simulink model "example_sdofplant"  (R2022b)
settings: Solver=VariableStepAuto  StartTime=0.0  StopTime=10.0  RelTol=1e-3
model workspace: external: MATLAB File exmaple_initdata.m (data not in the file)
undefined symbols (not defined in the file or in its folder): convertTo, datetime, Earth, F, Light, MIL, WGS84, WMM2020
libraries: aerolibconvert2 x5, aerolibasang x5, aerolibactuator x3, aerolibwind2 x3, aerolib6dof2 x1, aerolibatmos2 x1, aerolibgravity2 x1
settings Model: DataDictionary=example.sldd  Creator=zhanfuyu  LastModifiedBy=CETCA

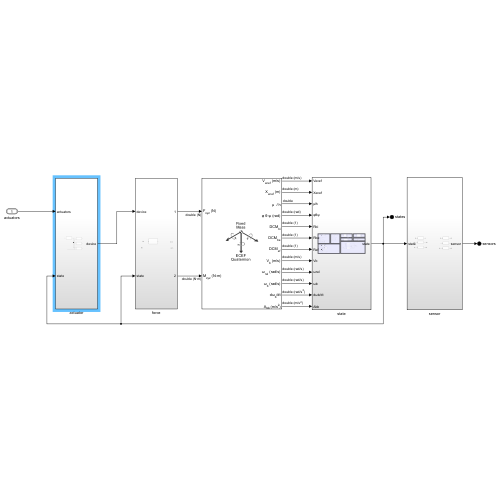
[thumbnail: Simulink's stored preview of the top-level diagram]
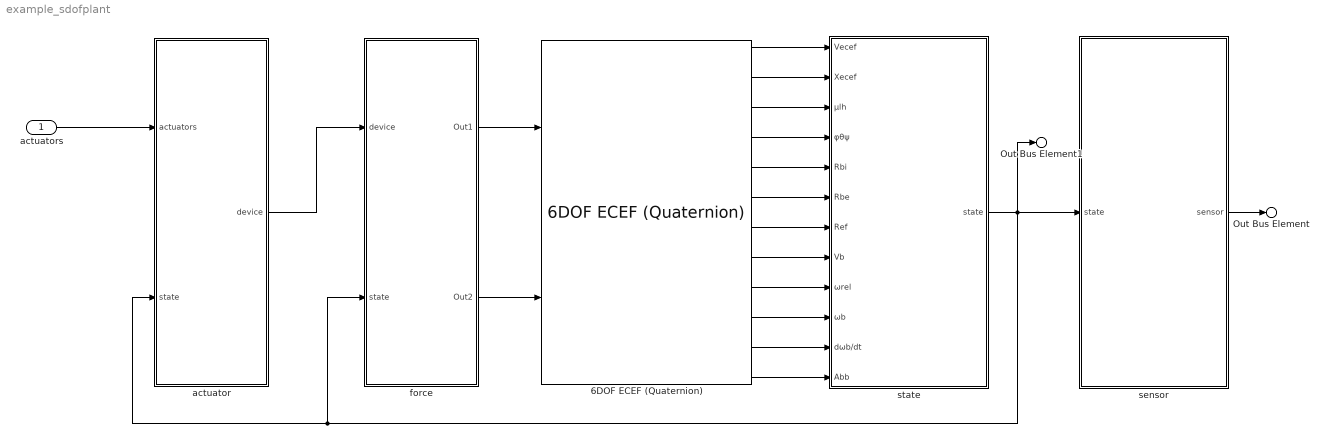
== system example_sdofplant ==
  actuators : Inport  OutDataTypeStr=Bus: actuator_outputs_s
  6DOF ECEF (Quaternion) : aerolib6dof2/6DOF ECEF (Quaternion)  units=Metric (MKS)  mtype=Fixed  xg_0=[0 0 0]  Vm_0=[0 0 0]  eul_0=[0 0 0]  pm_0=[0 0 0]  mass_0=1.0  mass_e=0.5  mass_f=2.0  inertia=eye(3)  inertia_e=eye(3)  inertia_f=2*eye(3)  vre_flag=on  abi_flag=off  ptype=Earth (WGS84)  R=6378137  F=1/298.257223563  w_E=7292115e-11  angle_in=Internal  LG0=0  quat_statename=''  pm_statename=''  Vm_statename=''  posECEF_statename=''  posECI_statename=''  LG_statename=''  mass_statename=''
  actuator : Subsystem
  force : Subsystem
  sensor : Subsystem
  state : Subsystem
  Out Bus Element : Outport  PortName=sensors
  Out Bus Element1 : Outport  Port=2  PortName=states
  wires:
  6DOF ECEF (Quaternion)/1 -> state/1(Vecef)
  6DOF ECEF (Quaternion)/2 -> state/2(Xecef)
  6DOF ECEF (Quaternion)/3 -> state/3(μlh)
  6DOF ECEF (Quaternion)/4 -> state/4(φθψ)
  6DOF ECEF (Quaternion)/5 -> state/5(Rbi)
  6DOF ECEF (Quaternion)/6 -> state/6(Rbe)
  6DOF ECEF (Quaternion)/7 -> state/7(Ref)
  6DOF ECEF (Quaternion)/8 -> state/8(Vb)
  6DOF ECEF (Quaternion)/9 -> state/9(ωrel)
  6DOF ECEF (Quaternion)/10 -> state/10(ωb)
  6DOF ECEF (Quaternion)/11 -> state/11(dωb/dt)
  6DOF ECEF (Quaternion)/12 -> state/12(Abb)
  state/1(state) -> Out Bus Element1/1, force/2(state), actuator/2(state), sensor/1(state)
  sensor/1(sensor) -> Out Bus Element/1
  force/1(Out1) -> 6DOF ECEF (Quaternion)/1
  force/2(Out2) -> 6DOF ECEF (Quaternion)/2
  actuator/1(device) -> force/1(device)
  actuators/1 -> actuator/1(actuators)

== system example_sdofplant/actuator ==
  Bus Element In1 : Inport  PortName=actuators  Element=output
  Bus Element In : Inport  Port=2  PortName=state
  Subsystem : Subsystem
  engine : Subsystem
  fixed wing : Subsystem
  rotor copter : Subsystem
  Bus Element Out : Outport  PortName=device
  wires:
  Bus Element In1/1 -> Subsystem/1(actuator_output)
  Subsystem/1(command) -> engine/1(command), rotor copter/1(command), fixed wing/1(command)
  Bus Element In/1 -> fixed wing/2(state), rotor copter/2(state), engine/2(state)

== system example_sdofplant/force ==
  Bus Element In1 : Inport  PortName=device
  Bus Element In : Inport  Port=2  PortName=state
  Aerodynamics : Subsystem
  Out1 : Outport
  Out2 : Outport  Port=2

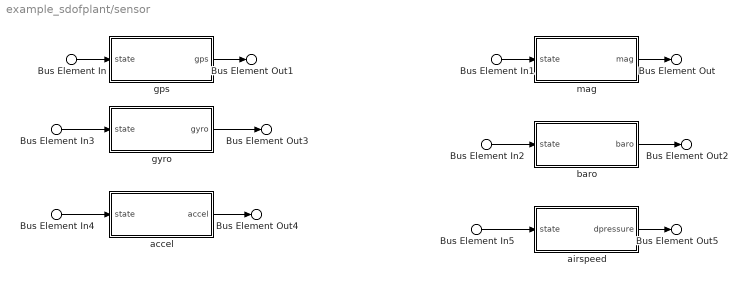
== system example_sdofplant/sensor ==
  Bus Element In{,1..5} (6 alike) : Inport  PortName=state
  accel : Subsystem
  airspeed : Subsystem
  baro : Subsystem
  gps : Subsystem
  gyro : Subsystem
  mag : Subsystem
  Bus Element Out1 : Outport  PortName=sensor  Element=gps
  Bus Element Out3 : Outport  PortName=sensor  Element=gyro
  Bus Element Out4 : Outport  PortName=sensor  Element=accel
  Bus Element Out : Outport  PortName=sensor  Element=mag
  Bus Element Out2 : Outport  PortName=sensor  Element=baro
  Bus Element Out5 : Outport  PortName=sensor  Element=dpressure
  wires:
  Bus Element In/1 -> gps/1(state)
  Bus Element In1/1 -> mag/1(state)
  mag/1(mag) -> Bus Element Out/1
  gps/1(gps) -> Bus Element Out1/1
  baro/1(baro) -> Bus Element Out2/1
  Bus Element In2/1 -> baro/1(state)
  Bus Element In3/1 -> gyro/1(state)
  gyro/1(gyro) -> Bus Element Out3/1
  Bus Element In4/1 -> accel/1(state)
  accel/1(accel) -> Bus Element Out4/1
  Bus Element In5/1 -> airspeed/1(state)
  airspeed/1(dpressure) -> Bus Element Out5/1

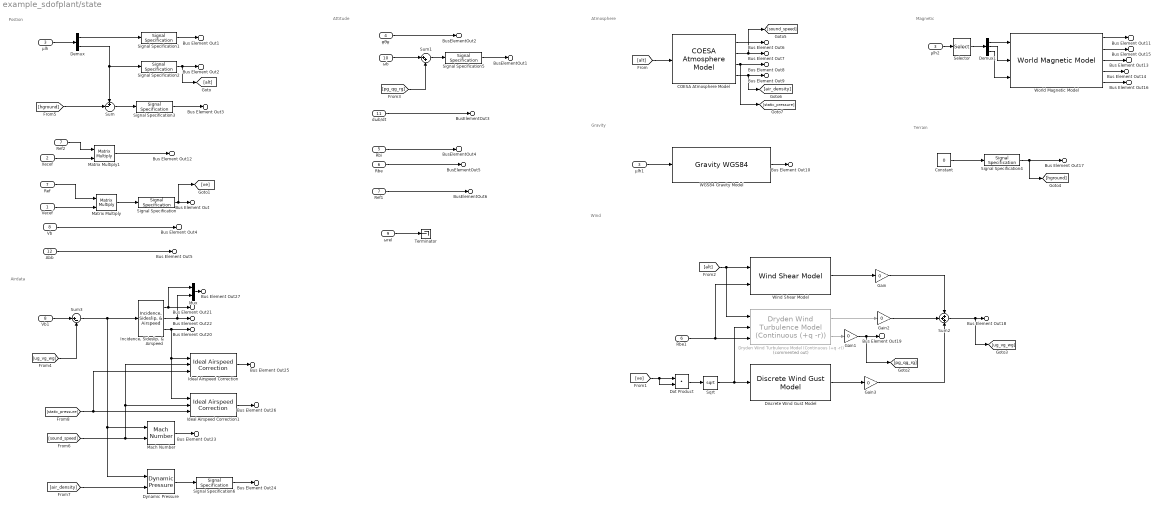
== system example_sdofplant/state ==
  note: Airdata
  note: Wind
  note: Terrain
  note: Magnetic
  note: Gravity
  note: Atmosphere
  note: Attitude
  note: Postion
  Vecef : Inport
  Xecef : Inport  Port=2
  μlh : Inport  Port=3
  φθψ : Inport  Port=4
  Rbi : Inport  Port=5
  Rbe : Inport  Port=6
  Ref : Inport  Port=7
  Vb : Inport  Port=8
  ωrel : Inport  Port=9
  ωb : Inport  Port=10
  dωb/dt : Inport  Port=11
  Abb : Inport  Port=12
  COESA Atmosphere Model : aerolibatmos2/COESA Atmosphere Model  units=Metric (MKS)  spec=1976 COESA-extended U.S. Standard Atmosphere  model=Profile  profile_var=High temperature  profile_percent=1%  profile_alt=5 km (16404 ft)  envelope_var=High temperature  envelope_percent=1%  action=Warning
  Constant : Constant  Value=0
  Demux : Demux  Outputs=[2 1]
  Demux1 : Demux  Outputs=3
  Discrete Wind Gust Model : aerolibwind2/Discrete Wind Gust Model  units=Metric (MKS)  Gx=on  Gy=on  Gz=on  t_0=5  d_m=[120 120 80]  v_m=[3.5 3.5 3.0]
  Dot Product : DotProduct  OutDataTypeStr=Inherit: Inherit via internal rule
  Dryden Wind Turbulence Model (Continuous (+q -r)) : aerolibwind2/Dryden Wind Turbulence Model  (Continuous (+q -r))  Commented=on  units=Metric (MKS)  spec=MIL-F-8785C  model=Continuous Dryden (+q -r)  W20=15  Wdeg=0  TurbProb=10^-2 - Light  L_high=533.4  Wingspan=10  ts=0.1  Seed=[23341 23342 23343 23344]  T_on=on
  Dynamic Pressure : aerolibasang/Dynamic Pressure
  Gain{,1..3} (4 alike) : Gain  Gain=0
  Ideal Airspeed Correction : aerolibasang/Ideal Airspeed Correction  units=Metric (MKS)  vel_in=TAS  vel_out_tas=CAS  vel_out_eas=TAS  vel_out_cas=TAS  method=Table Lookup  SubOnly=off  action=None
  Ideal Airspeed Correction1 : aerolibasang/Ideal Airspeed Correction  units=Metric (MKS)  vel_in=TAS  vel_out_tas=EAS  vel_out_eas=TAS  vel_out_cas=TAS  method=Table Lookup  SubOnly=off  action=None
  "Incidence, Sideslip, & Airspeed" : aerolibasang/Incidence, Sideslip, & Airspeed
  Mach Number : aerolibasang/Mach Number
  Matrix Multiply : Product  Multiplication=Matrix(*)
  Matrix Multiply1 : Product  Multiplication=Matrix(*)
  Mux : Mux  Inputs=2
  Rbe1 : InportShadow  Port=6
  Ref1 : InportShadow  Port=7
  Ref2 : InportShadow  Port=7
  Selector : Selector  InputPortWidth=3  IndexOptions=Index vector (dialog)  Indices=[3 1 2]  OutputSizes=1
  Signal Specification : SignalSpecification  Unit=m/s
  Signal Specification1 : SignalSpecification  Unit=deg
  Signal Specification2 : SignalSpecification  Unit=m
  Signal Specification3 : SignalSpecification  Unit=m
  Signal Specification4 : SignalSpecification  Unit=m
  Signal Specification5 : SignalSpecification  Unit=rad/s
  Signal Specification6 : SignalSpecification  Unit=Pa
  Sqrt : Sqrt
  Sum : Sum  Inputs=+-|
  Sum1 : Sum  Inputs=|++
  Sum2 : Sum  Inputs=+++
  Sum3 : Sum  Inputs=|+-
  Terminator : Terminator
  Vb1 : InportShadow  Port=8
  "WGS84 Gravity Model  " : GravityWGS84
  Wind Shear Model : aerolibwind2/Wind Shear Model  units=Metric (MKS)  phase=Category C - Terminal Flight Phase  W_20=15  Wdeg=0
  World Magnetic Model : aerolibgravity2/World Magnetic Model  model=WMM2020 (2020-2025)  customFile='WMM2020.COF'  units=Metric (MKS)  time_in=off  month=January  day=1  year=2020  action=Error  h_out=on  dec_out=on  inc_out=on  ti_out=on
  μlh1 : InportShadow  Port=3
  μlh2 : InportShadow  Port=3
  Bus Element Out1 : Outport  PortName=state  Element=aircraft.position.lat_lon
  Bus Element Out2 : Outport  PortName=state  Element=aircraft.position.alt
  Bus Element Out3 : Outport  PortName=state  Element=aircraft.position.agl
  Bus Element Out12 : Outport  PortName=state  Element=aircraft.position.pn_pe_pd
  Bus Element Out : Outport  PortName=state  Element=aircraft.position.vn_ve_vd
  Bus Element Out4 : Outport  PortName=state  Element=aircraft.position.ub_vb_wb
  Bus Element Out5 : Outport  PortName=state  Element=aircraft.position.ax_ay_az
  BusElementOut2 : Outport  PortName=state  Element=aircraft.attitude.phi_theta_psi
  BusElementOut1 : Outport  PortName=state  Element=aircraft.attitude.p_q_r
  BusElementOut3 : Outport  PortName=state  Element=aircraft.attitude.pdot_qdot_rdot
  BusElementOut4 : Outport  PortName=state  Element=aircraft.attitude.Rbi
  BusElementOut5 : Outport  PortName=state  Element=aircraft.attitude.Rbe
  BusElementOut6 : Outport  PortName=state  Element=aircraft.attitude.Ref
  Bus Element Out20 : Outport  PortName=state  Element=aircraft.airdata.airspeed
  Bus Element Out21 : Outport  PortName=state  Element=aircraft.airdata.alpha
  Bus Element Out22 : Outport  PortName=state  Element=aircraft.airdata.bata
  Bus Element Out23 : Outport  PortName=state  Element=aircraft.airdata.mach
  Bus Element Out24 : Outport  PortName=state  Element=aircraft.airdata.qbar
  Bus Element Out25 : Outport  PortName=state  Element=aircraft.airdata.airspeed_cali
  Bus Element Out26 : Outport  PortName=state  Element=aircraft.airdata.airspeed_equ
  Bus Element Out27 : Outport  PortName=state  Element=aircraft.airdata.alpha_beta
  Bus Element Out6 : Outport  PortName=state  Element=environ.atmosphere.temperature
  Bus Element Out7 : Outport  PortName=state  Element=environ.atmosphere.soundspeed
  Bus Element Out8 : Outport  PortName=state  Element=environ.atmosphere.pressure
  Bus Element Out9 : Outport  PortName=state  Element=environ.atmosphere.density
  Bus Element Out10 : Outport  PortName=state  Element=environ.gravity.xyz
  Bus Element Out11 : Outport  PortName=state  Element=environ.magnetic.xyz
  Bus Element Out13 : Outport  PortName=state  Element=environ.magnetic.declination
  Bus Element Out14 : Outport  PortName=state  Element=environ.magnetic.inclination
  Bus Element Out15 : Outport  PortName=state  Element=environ.magnetic.hor_intensity
  Bus Element Out16 : Outport  PortName=state  Element=environ.magnetic.total_intensity
  Bus Element Out17 : Outport  PortName=state  Element=environ.terrain.hground
  Bus Element Out18 : Outport  PortName=state  Element=environ.wind.ug_vg_wg
  Bus Element Out19 : Outport  PortName=state  Element=environ.wind.pg_qg_rg
  wires:
  Ref/1 -> Matrix Multiply/1
  Vecef/1 -> Matrix Multiply/2
  Matrix Multiply/1 -> Signal Specification/1
  Signal Specification/1 -> [ve], Bus Element Out/1
  μlh/1 -> Demux/1
  Demux/1 -> Signal Specification1/1
  Signal Specification1/1 -> Bus Element Out1/1
  Demux/2 -> Signal Specification2/1, Sum/1
  Signal Specification2/1 -> [alt], Bus Element Out2/1
  Sum/1 -> Signal Specification3/1
  Signal Specification3/1 -> Bus Element Out3/1
  [hground] -> Sum/2
  Vb/1 -> Bus Element Out4/1
  Abb/1 -> Bus Element Out5/1
  φθψ/1 -> BusElementOut2/1
  Rbi/1 -> BusElementOut4/1
  Rbe/1 -> BusElementOut5/1
  Ref1/1 -> BusElementOut6/1
  ωb/1 -> Sum1/1
  Sum1/1 -> Signal Specification5/1
  [pg_qg_rg] -> Sum1/2
  dωb/dt/1 -> BusElementOut3/1
  ωrel/1 -> Terminator/1
  Xecef/1 -> Matrix Multiply1/2
  Ref2/1 -> Matrix Multiply1/1
  Matrix Multiply1/1 -> Bus Element Out12/1
  [alt] -> COESA Atmosphere Model/1
  COESA Atmosphere Model/1 -> Bus Element Out6/1
  COESA Atmosphere Model/2 -> [sound_speed], Bus Element Out7/1
  COESA Atmosphere Model/3 -> [static_pressure], Bus Element Out8/1
  COESA Atmosphere Model/4 -> [air_density], Bus Element Out9/1
  μlh1/1 -> "WGS84 Gravity Model  "/1
  "WGS84 Gravity Model  "/1 -> Bus Element Out10/1
  μlh2/1 -> Selector/1
  Selector/1 -> Demux1/1
  Demux1/1 -> World Magnetic Model/1
  Demux1/2 -> World Magnetic Model/2
  Demux1/3 -> World Magnetic Model/3
  World Magnetic Model/1 -> Bus Element Out11/1
  World Magnetic Model/3 -> Bus Element Out13/1
  World Magnetic Model/4 -> Bus Element Out14/1
  World Magnetic Model/2 -> Bus Element Out15/1
  World Magnetic Model/5 -> Bus Element Out16/1
  Constant/1 -> Signal Specification4/1
  Signal Specification4/1 -> [hground], Bus Element Out17/1
  Dryden Wind Turbulence Model (Continuous (+q -r))/1 -> Gain2/1
  Discrete Wind Gust Model/1 -> Gain3/1
  Dryden Wind Turbulence Model (Continuous (+q -r))/2 -> Gain1/1
  Rbe1/1 -> Wind Shear Model/2, Dryden Wind Turbulence Model (Continuous (+q -r))/3
  [alt] -> Wind Shear Model/1, Dryden Wind Turbulence Model (Continuous (+q -r))/1
  [ve] -> Dot Product/2, Dot Product/1
  Dot Product/1 -> Sqrt/1
  Sqrt/1 -> Dryden Wind Turbulence Model (Continuous (+q -r))/2, Discrete Wind Gust Model/1
  Sum2/1 -> [ug_vg_wg], Bus Element Out18/1
  Wind Shear Model/1 -> Gain/1
  Gain1/1 -> [pg_qg_rg], Bus Element Out19/1
  Vb1/1 -> Sum3/1
  [ug_vg_wg] -> Sum3/2
  Sum3/1 -> "Incidence, Sideslip, & Airspeed"/1, Dynamic Pressure/1, Mach Number/1
  "Incidence, Sideslip, & Airspeed"/3 -> Ideal Airspeed Correction/1, Ideal Airspeed Correction1/1, Bus Element Out20/1
  "Incidence, Sideslip, & Airspeed"/2 -> Mux/2, Bus Element Out22/1
  "Incidence, Sideslip, & Airspeed"/1 -> Mux/1, Bus Element Out21/1
  [sound_speed] -> Ideal Airspeed Correction1/2, Ideal Airspeed Correction/2, Mach Number/2
  Mach Number/1 -> Bus Element Out23/1
  Dynamic Pressure/1 -> Signal Specification6/1
  [air_density] -> Dynamic Pressure/2
  [static_pressure] -> Ideal Airspeed Correction/3, Ideal Airspeed Correction1/3
  Ideal Airspeed Correction/1 -> Bus Element Out25/1
  Ideal Airspeed Correction1/1 -> Bus Element Out26/1
  Mux/1 -> Bus Element Out27/1
  Gain/1 -> Sum2/1
  Gain2/1 -> Sum2/2
  Gain3/1 -> Sum2/3
  Signal Specification5/1 -> BusElementOut1/1
  Signal Specification6/1 -> Bus Element Out24/1

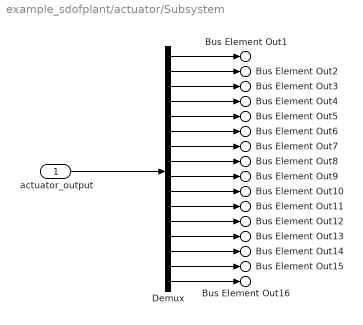
== system example_sdofplant/actuator/Subsystem ==
  actuator_output : Inport
  Demux : Demux  Outputs=16
  Bus Element Out1 : Outport  PortName=command  Element=pwm1
  Bus Element Out2 : Outport  PortName=command  Element=pwm2
  Bus Element Out3 : Outport  PortName=command  Element=pwm3
  Bus Element Out4 : Outport  PortName=command  Element=pwm4
  Bus Element Out5 : Outport  PortName=command  Element=pwm5
  Bus Element Out6 : Outport  PortName=command  Element=pwm6
  Bus Element Out7 : Outport  PortName=command  Element=pwm7
  Bus Element Out8 : Outport  PortName=command  Element=pwm8
  Bus Element Out9 : Outport  PortName=command  Element=pwm9
  Bus Element Out10 : Outport  PortName=command  Element=pwm10
  Bus Element Out11 : Outport  PortName=command  Element=pwm11
  Bus Element Out12 : Outport  PortName=command  Element=pwm12
  Bus Element Out13 : Outport  PortName=command  Element=pwm13
  Bus Element Out14 : Outport  PortName=command  Element=pwm14
  Bus Element Out15 : Outport  PortName=command  Element=pwm15
  Bus Element Out16 : Outport  PortName=command  Element=pwm16
  wires:
  actuator_output/1 -> Demux/1
  Demux/1 -> Bus Element Out1/1
  Demux/2 -> Bus Element Out2/1
  Demux/3 -> Bus Element Out3/1
  Demux/4 -> Bus Element Out4/1
  Demux/5 -> Bus Element Out5/1
  Demux/6 -> Bus Element Out6/1
  Demux/7 -> Bus Element Out7/1
  Demux/8 -> Bus Element Out8/1
  Demux/9 -> Bus Element Out9/1
  Demux/10 -> Bus Element Out10/1
  Demux/11 -> Bus Element Out11/1
  Demux/12 -> Bus Element Out12/1
  Demux/13 -> Bus Element Out13/1
  Demux/14 -> Bus Element Out14/1
  Demux/15 -> Bus Element Out15/1
  Demux/16 -> Bus Element Out16/1

== system example_sdofplant/actuator/engine ==
  Bus Element In : Inport  PortName=command
  Bus Element In1 : Inport  Port=2  PortName=state
  Linear Second-Order Actuator : aerolibactuator/Linear Second-Order Actuator  wn_fin=1  z_fin=0.3  fin_act_0=0  fin_act_vel=0
  Bus Element Out : Outport  PortName=OutBus  Element=signal1

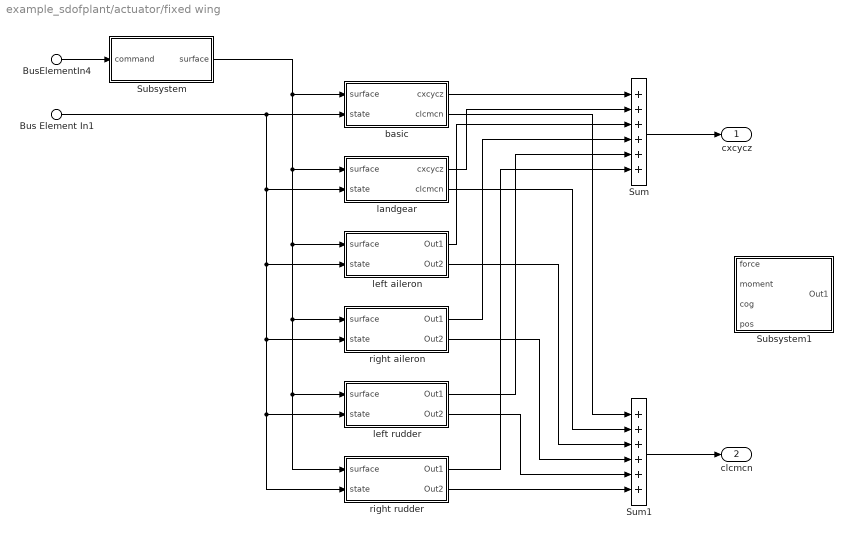
== system example_sdofplant/actuator/fixed wing ==
  BusElementIn4 : Inport  PortName=command
  Bus Element In1 : Inport  Port=2  PortName=state
  Subsystem : Subsystem
  Subsystem1 : Subsystem
  Sum : Sum  Inputs=6
  Sum1 : Sum  Inputs=6
  basic : Subsystem
  landgear : Subsystem
  left aileron : Subsystem
  left rudder : Subsystem
  right aileron : Subsystem
  right rudder : Subsystem
  cxcycz : Outport
  clcmcn : Outport  Port=2
  wires:
  BusElementIn4/1 -> Subsystem/1(command)
  left aileron/1(Out1) -> Sum/3
  right aileron/1(Out1) -> Sum/4
  landgear/1(cxcycz) -> Sum/2
  left rudder/1(Out1) -> Sum/5
  basic/1(cxcycz) -> Sum/1
  right rudder/1(Out1) -> Sum/6
  Sum/1 -> cxcycz/1
  Subsystem/1(surface) -> landgear/1(surface), right rudder/1(surface), left rudder/1(surface), right aileron/1(surface), left aileron/1(surface), basic/1(surface)
  Bus Element In1/1 -> basic/2(state), landgear/2(state), right rudder/2(state), left rudder/2(state), right aileron/2(state), left aileron/2(state)
  basic/2(clcmcn) -> Sum1/1
  landgear/2(clcmcn) -> Sum1/2
  Sum1/1 -> clcmcn/1
  left aileron/2(Out2) -> Sum1/3
  right aileron/2(Out2) -> Sum1/4
  left rudder/2(Out2) -> Sum1/5
  right rudder/2(Out2) -> Sum1/6

== system example_sdofplant/actuator/rotor copter ==
  Bus Element In : Inport  PortName=command  Element=pwm1
  Bus Element In2 : Inport  PortName=command  Element=pwm2
  Bus Element In3 : Inport  PortName=command  Element=pwm3
  Bus Element In4 : Inport  PortName=command  Element=pwm4
  Bus Element In1 : Inport  Port=2  PortName=state
  Constant : Constant  Value=1000
  Gain : Gain  Gain=1/1000
  Linear Second-Order Actuator : aerolibactuator/Linear Second-Order Actuator  wn_fin=1  z_fin=0.3  fin_act_0=0  fin_act_vel=0
  Mux : Mux
  Saturation : Saturate  UpperLimit=1  LowerLimit=0
  Sum : Sum  Inputs=|+-
  Bus Element Out : Outport  PortName=rotor  Element=rpm
  wires:
  Bus Element In3/1 -> Mux/3
  Bus Element In2/1 -> Mux/2
  Bus Element In4/1 -> Mux/4
  Bus Element In/1 -> Mux/1
  Mux/1 -> Sum/1
  Constant/1 -> Sum/2
  Sum/1 -> Gain/1
  Gain/1 -> Saturation/1
  Saturation/1 -> Linear Second-Order Actuator/1
  Linear Second-Order Actuator/1 -> Bus Element Out/1

== system example_sdofplant/force/Aerodynamics ==
  In1 : Inport
  Out1 : Outport
  wires:
  In1/1 -> Out1/1

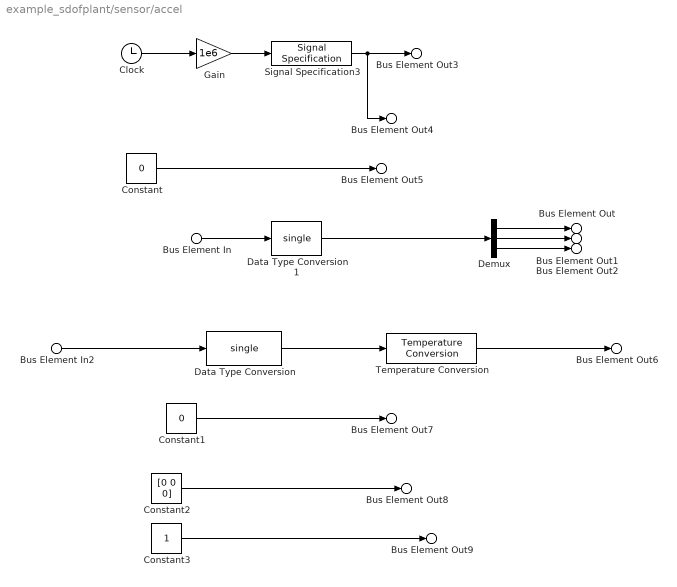
== system example_sdofplant/sensor/accel ==
  Bus Element In2 : Inport  PortName=state  Element=environ.atmosphere.temperature
  Bus Element In : Inport  PortName=state  Element=aircraft.position.ax_ay_az
  Clock : Clock
  Constant : Constant  Value=0  OutDataTypeStr=uint32
  Constant1 : Constant  Value=0  OutDataTypeStr=uint32
  Constant2 : Constant  Value=[0 0 0]  OutDataTypeStr=uint8
  Constant3 : Constant  OutDataTypeStr=uint8
  Data Type Conversion : DataTypeConversion  OutDataTypeStr=single  SaturateOnIntegerOverflow=off  RndMeth=Floor
  Data Type Conversion1 : DataTypeConversion  OutDataTypeStr=single  SaturateOnIntegerOverflow=off  RndMeth=Floor
  Demux : Demux  Outputs=3
  Gain : Gain  Gain=1e6  OutDataTypeStr=uint64
  Signal Specification3 : SignalSpecification  Unit=µs
  Temperature Conversion : aerolibconvert2/Temperature Conversion  IU=K  OU=C
  Bus Element Out3 : Outport  PortName=accel  Element=timestamp
  Bus Element Out4 : Outport  PortName=accel  Element=timestamp_sample
  Bus Element Out5 : Outport  PortName=accel  Element=device_id
  Bus Element Out : Outport  PortName=accel  Element=x
  Bus Element Out1 : Outport  PortName=accel  Element=y
  Bus Element Out2 : Outport  PortName=accel  Element=z
  Bus Element Out6 : Outport  PortName=accel  Element=temperature
  Bus Element Out7 : Outport  PortName=accel  Element=error_count
  Bus Element Out8 : Outport  PortName=accel  Element=clip_counter
  Bus Element Out9 : Outport  PortName=accel  Element=samples
  wires:
  Constant3/1 -> Bus Element Out9/1
  Constant2/1 -> Bus Element Out8/1
  Bus Element In/1 -> Data Type Conversion1/1
  Demux/1 -> Bus Element Out/1
  Demux/2 -> Bus Element Out1/1
  Demux/3 -> Bus Element Out2/1
  Clock/1 -> Gain/1
  Signal Specification3/1 -> Bus Element Out4/1, Bus Element Out3/1
  Gain/1 -> Signal Specification3/1
  Constant/1 -> Bus Element Out5/1
  Constant1/1 -> Bus Element Out7/1
  Bus Element In2/1 -> Data Type Conversion/1
  Temperature Conversion/1 -> Bus Element Out6/1
  Data Type Conversion/1 -> Temperature Conversion/1
  Data Type Conversion1/1 -> Demux/1

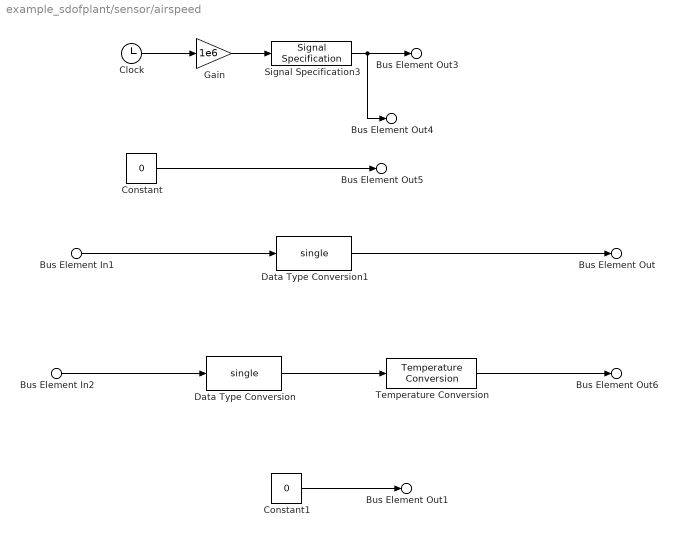
== system example_sdofplant/sensor/airspeed ==
  Bus Element In2 : Inport  PortName=state  Element=environ.atmosphere.temperature
  Bus Element In1 : Inport  PortName=state  Element=aircraft.airdata.qbar
  Clock : Clock
  Constant : Constant  Value=0  OutDataTypeStr=uint32
  Constant1 : Constant  Value=0  OutDataTypeStr=uint32
  Data Type Conversion : DataTypeConversion  OutDataTypeStr=single  SaturateOnIntegerOverflow=off  RndMeth=Floor
  Data Type Conversion1 : DataTypeConversion  OutDataTypeStr=single  SaturateOnIntegerOverflow=off  RndMeth=Floor
  Gain : Gain  Gain=1e6  OutDataTypeStr=uint64
  Signal Specification3 : SignalSpecification  Unit=µs
  Temperature Conversion : aerolibconvert2/Temperature Conversion  IU=K  OU=C
  Bus Element Out3 : Outport  PortName=dpressure  Element=timestamp
  Bus Element Out4 : Outport  PortName=dpressure  Element=timestamp_sample
  Bus Element Out5 : Outport  PortName=dpressure  Element=device_id
  Bus Element Out : Outport  PortName=dpressure  Element=differential_pressure_pa
  Bus Element Out6 : Outport  PortName=dpressure  Element=temperature
  Bus Element Out1 : Outport  PortName=dpressure  Element=error_count
  wires:
  Data Type Conversion1/1 -> Bus Element Out/1
  Bus Element In1/1 -> Data Type Conversion1/1
  Data Type Conversion/1 -> Temperature Conversion/1
  Temperature Conversion/1 -> Bus Element Out6/1
  Bus Element In2/1 -> Data Type Conversion/1
  Constant/1 -> Bus Element Out5/1
  Gain/1 -> Signal Specification3/1
  Signal Specification3/1 -> Bus Element Out3/1, Bus Element Out4/1
  Clock/1 -> Gain/1
  Constant1/1 -> Bus Element Out1/1

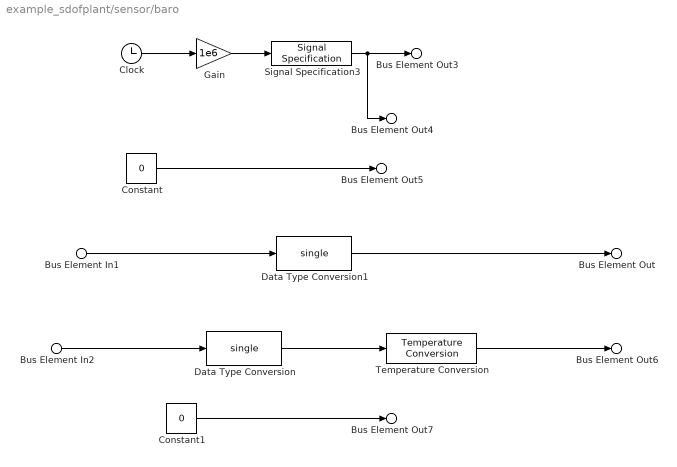
== system example_sdofplant/sensor/baro ==
  Bus Element In2 : Inport  PortName=state  Element=environ.atmosphere.temperature
  Bus Element In1 : Inport  PortName=state  Element=environ.atmosphere.pressure
  Clock : Clock
  Constant : Constant  Value=0  OutDataTypeStr=uint32
  Constant1 : Constant  Value=0  OutDataTypeStr=uint32
  Data Type Conversion : DataTypeConversion  OutDataTypeStr=single  SaturateOnIntegerOverflow=off  RndMeth=Floor
  Data Type Conversion1 : DataTypeConversion  OutDataTypeStr=single  SaturateOnIntegerOverflow=off  RndMeth=Floor
  Gain : Gain  Gain=1e6  OutDataTypeStr=uint64
  Signal Specification3 : SignalSpecification  Unit=µs
  Temperature Conversion : aerolibconvert2/Temperature Conversion  IU=K  OU=C
  Bus Element Out3 : Outport  PortName=baro  Element=timestamp
  Bus Element Out4 : Outport  PortName=baro  Element=timestamp_sample
  Bus Element Out5 : Outport  PortName=baro  Element=device_id
  Bus Element Out : Outport  PortName=baro  Element=pressure
  Bus Element Out6 : Outport  PortName=baro  Element=temperature
  Bus Element Out7 : Outport  PortName=baro  Element=error_count
  wires:
  Clock/1 -> Gain/1
  Signal Specification3/1 -> Bus Element Out4/1, Bus Element Out3/1
  Gain/1 -> Signal Specification3/1
  Constant/1 -> Bus Element Out5/1
  Constant1/1 -> Bus Element Out7/1
  Bus Element In2/1 -> Data Type Conversion/1
  Temperature Conversion/1 -> Bus Element Out6/1
  Data Type Conversion/1 -> Temperature Conversion/1
  Bus Element In1/1 -> Data Type Conversion1/1
  Data Type Conversion1/1 -> Bus Element Out/1

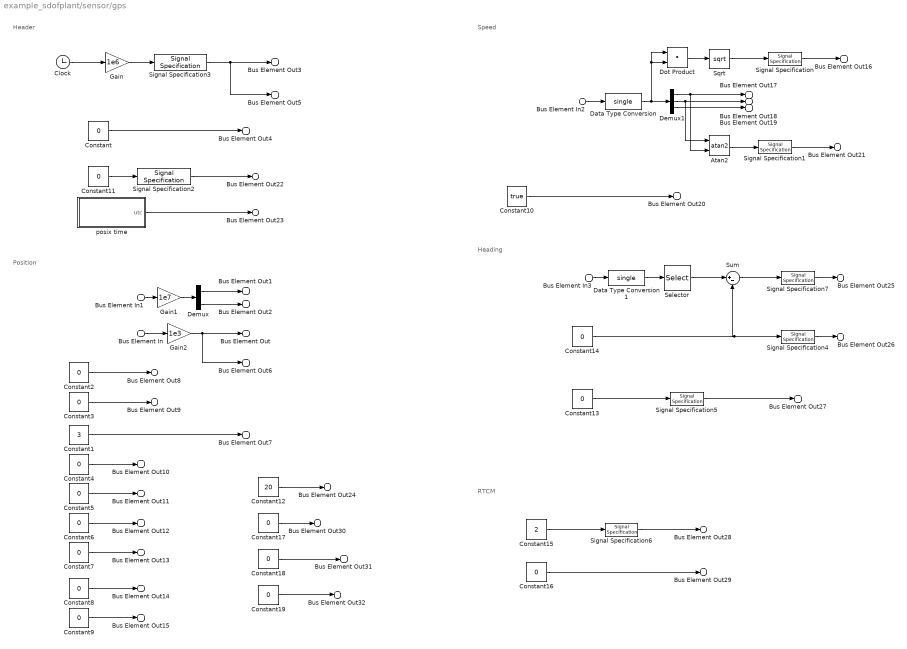
== system example_sdofplant/sensor/gps ==
  note: RTCM
  note: Heading
  note: Speed
  note: Header
  note: Position
  Bus Element In : Inport  PortName=state  Element=aircraft.position.alt
  Bus Element In1 : Inport  PortName=state  Element=aircraft.position.lat_lon
  Bus Element In2 : Inport  PortName=state  Element=aircraft.position.vn_ve_vd
  Bus Element In3 : Inport  PortName=state  Element=aircraft.attitude.phi_theta_psi
  Atan2 : Trigonometry  Operator=atan2
  Clock : Clock
  Constant : Constant  Value=0  OutDataTypeStr=uint32
  Constant1 : Constant  Value=3  OutDataTypeStr=uint8
  Constant10 : Constant  Value=true  OutDataTypeStr=boolean
  Constant11 : Constant  Value=0  OutDataTypeStr=uint32
  Constant12 : Constant  Value=20  OutDataTypeStr=uint8
  Constant{2..7,13..14} (8 alike) : Constant  Value=0  OutDataTypeStr=single
  Constant15 : Constant  Value=2  OutDataTypeStr=single
  Constant16 : Constant  Value=0  OutDataTypeStr=uint8
  Constant17 : Constant  Value=0  OutDataTypeStr=uint8
  Constant18 : Constant  Value=0  OutDataTypeStr=int32
  Constant19 : Constant  Value=0  OutDataTypeStr=uint8
  Constant8 : Constant  Value=0  OutDataTypeStr=int32
  Constant9 : Constant  Value=0  OutDataTypeStr=uint16
  Data Type Conversion : DataTypeConversion  OutDataTypeStr=single  SaturateOnIntegerOverflow=off  RndMeth=Floor
  Data Type Conversion1 : DataTypeConversion  OutDataTypeStr=single  SaturateOnIntegerOverflow=off  RndMeth=Floor
  Demux : Demux  Outputs=2
  Demux1 : Demux  Outputs=3
  Dot Product : DotProduct  OutDataTypeStr=Inherit: Inherit via internal rule
  Gain : Gain  Gain=1e6  OutDataTypeStr=uint64
  Gain1 : Gain  Gain=1e7  OutDataTypeStr=int32
  Gain2 : Gain  Gain=1e3  OutDataTypeStr=int32
  Selector : Selector  InputPortWidth=3  IndexOptions=Index vector (dialog)  Indices=3  OutputSizes=1
  Signal Specification : SignalSpecification  Unit=m/s
  Signal Specification{1,4..5,7} (4 alike) : SignalSpecification  Unit=rad
  Signal Specification2 : SignalSpecification  Unit=ms
  Signal Specification3 : SignalSpecification  Unit=µs
  Signal Specification6 : SignalSpecification  Unit=Hz
  Sqrt : Sqrt
  Sum : Sum  Inputs=|+-
  posix time : Subsystem
  Bus Element Out3 : Outport  PortName=gps  Element=timestamp
  Bus Element Out5 : Outport  PortName=gps  Element=timestamp_sample
  Bus Element Out4 : Outport  PortName=gps  Element=device_id
  Bus Element Out1 : Outport  PortName=gps  Element=lat
  Bus Element Out2 : Outport  PortName=gps  Element=lon
  Bus Element Out : Outport  PortName=gps  Element=alt
  Bus Element Out6 : Outport  PortName=gps  Element=alt_ellipsoid
  Bus Element Out8 : Outport  PortName=gps  Element=s_variance_m_s
  Bus Element Out9 : Outport  PortName=gps  Element=c_variance_rad
  Bus Element Out7 : Outport  PortName=gps  Element=fix_type
  Bus Element Out10 : Outport  PortName=gps  Element=eph
  Bus Element Out11 : Outport  PortName=gps  Element=epv
  Bus Element Out12 : Outport  PortName=gps  Element=hdop
  Bus Element Out13 : Outport  PortName=gps  Element=vdop
  Bus Element Out14 : Outport  PortName=gps  Element=noise_per_ms
  Bus Element Out15 : Outport  PortName=gps  Element=automatic_gain_control
  Bus Element Out30 : Outport  PortName=gps  Element=jamming_state
  Bus Element Out31 : Outport  PortName=gps  Element=jamming_indicator
  Bus Element Out32 : Outport  PortName=gps  Element=spoofing_state
  Bus Element Out16 : Outport  PortName=gps  Element=vel_m_s
  Bus Element Out17 : Outport  PortName=gps  Element=vel_n_m_s
  Bus Element Out18 : Outport  PortName=gps  Element=vel_e_m_s
  Bus Element Out19 : Outport  PortName=gps  Element=vel_d_m_s
  Bus Element Out21 : Outport  PortName=gps  Element=cog_rad
  Bus Element Out20 : Outport  PortName=gps  Element=vel_ned_valid
  Bus Element Out22 : Outport  PortName=gps  Element=timestamp_time_relative
  Bus Element Out23 : Outport  PortName=gps  Element=time_utc_usec
  Bus Element Out24 : Outport  PortName=gps  Element=satellites_used
  Bus Element Out25 : Outport  PortName=gps  Element=heading
  Bus Element Out26 : Outport  PortName=gps  Element=heading_offset
  Bus Element Out27 : Outport  PortName=gps  Element=heading_accuracy
  Bus Element Out28 : Outport  PortName=gps  Element=rtcm_injection_rate
  Bus Element Out29 : Outport  PortName=gps  Element=selected_rtcm_instance
  wires:
  Bus Element In/1 -> Gain2/1
  Bus Element In1/1 -> Gain1/1
  Demux/1 -> Bus Element Out1/1
  Demux/2 -> Bus Element Out2/1
  Clock/1 -> Gain/1
  Gain/1 -> Signal Specification3/1
  Constant/1 -> Bus Element Out4/1
  Gain1/1 -> Demux/1
  Gain2/1 -> Bus Element Out6/1, Bus Element Out/1
  Constant1/1 -> Bus Element Out7/1
  Constant2/1 -> Bus Element Out8/1
  Constant3/1 -> Bus Element Out9/1
  Constant4/1 -> Bus Element Out10/1
  Constant5/1 -> Bus Element Out11/1
  Constant7/1 -> Bus Element Out13/1
  Constant6/1 -> Bus Element Out12/1
  Constant9/1 -> Bus Element Out15/1
  Constant8/1 -> Bus Element Out14/1
  Bus Element In2/1 -> Data Type Conversion/1
  Demux1/1 -> Atan2/2, Bus Element Out17/1
  Demux1/2 -> Atan2/1, Bus Element Out18/1
  Demux1/3 -> Bus Element Out19/1
  Constant10/1 -> Bus Element Out20/1
  Atan2/1 -> Signal Specification1/1
  Sqrt/1 -> Signal Specification/1
  Dot Product/1 -> Sqrt/1
  Data Type Conversion/1 -> Demux1/1, Dot Product/1, Dot Product/2
  Signal Specification/1 -> Bus Element Out16/1
  Signal Specification1/1 -> Bus Element Out21/1
  Constant12/1 -> Bus Element Out24/1
  Bus Element In3/1 -> Data Type Conversion1/1
  Constant14/1 -> Sum/2, Signal Specification4/1
  Selector/1 -> Sum/1
  Constant13/1 -> Signal Specification5/1
  Sum/1 -> Signal Specification7/1
  Constant15/1 -> Signal Specification6/1
  Constant16/1 -> Bus Element Out29/1
  Constant11/1 -> Signal Specification2/1
  posix time/1(utc) -> Bus Element Out23/1
  Signal Specification2/1 -> Bus Element Out22/1
  Signal Specification3/1 -> Bus Element Out5/1, Bus Element Out3/1
  Signal Specification4/1 -> Bus Element Out26/1
  Signal Specification5/1 -> Bus Element Out27/1
  Signal Specification6/1 -> Bus Element Out28/1
  Constant17/1 -> Bus Element Out30/1
  Constant18/1 -> Bus Element Out31/1
  Constant19/1 -> Bus Element Out32/1
  Signal Specification7/1 -> Bus Element Out25/1
  Data Type Conversion1/1 -> Selector/1

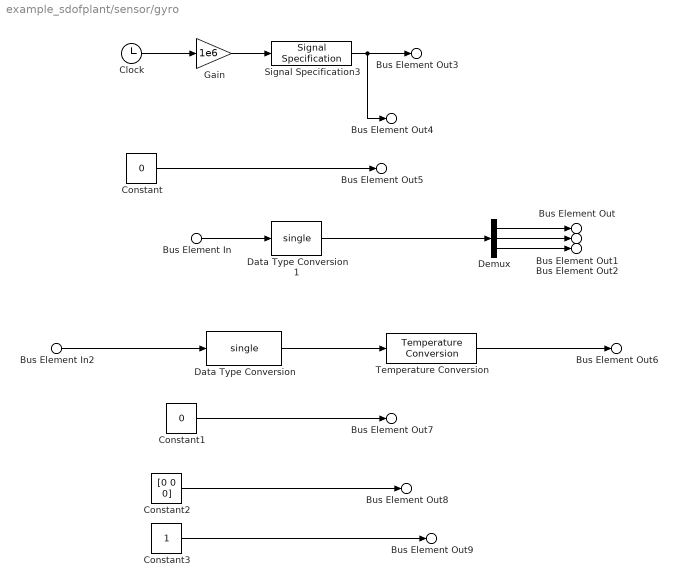
== system example_sdofplant/sensor/gyro ==
  Bus Element In2 : Inport  PortName=state  Element=environ.atmosphere.temperature
  Bus Element In : Inport  PortName=state  Element=aircraft.attitude.p_q_r
  Clock : Clock
  Constant : Constant  Value=0  OutDataTypeStr=uint32
  Constant1 : Constant  Value=0  OutDataTypeStr=uint32
  Constant2 : Constant  Value=[0 0 0]  OutDataTypeStr=uint8
  Constant3 : Constant  OutDataTypeStr=uint8
  Data Type Conversion : DataTypeConversion  OutDataTypeStr=single  SaturateOnIntegerOverflow=off  RndMeth=Floor
  Data Type Conversion1 : DataTypeConversion  OutDataTypeStr=single  SaturateOnIntegerOverflow=off  RndMeth=Floor
  Demux : Demux  Outputs=3
  Gain : Gain  Gain=1e6  OutDataTypeStr=uint64
  Signal Specification3 : SignalSpecification  Unit=µs
  Temperature Conversion : aerolibconvert2/Temperature Conversion  IU=K  OU=C
  Bus Element Out3 : Outport  PortName=gyro  Element=timestamp
  Bus Element Out4 : Outport  PortName=gyro  Element=timestamp_sample
  Bus Element Out5 : Outport  PortName=gyro  Element=device_id
  Bus Element Out : Outport  PortName=gyro  Element=x
  Bus Element Out1 : Outport  PortName=gyro  Element=y
  Bus Element Out2 : Outport  PortName=gyro  Element=z
  Bus Element Out6 : Outport  PortName=gyro  Element=temperature
  Bus Element Out7 : Outport  PortName=gyro  Element=error_count
  Bus Element Out8 : Outport  PortName=gyro  Element=clip_counter
  Bus Element Out9 : Outport  PortName=gyro  Element=samples
  wires:
  Data Type Conversion1/1 -> Demux/1
  Data Type Conversion/1 -> Temperature Conversion/1
  Temperature Conversion/1 -> Bus Element Out6/1
  Bus Element In2/1 -> Data Type Conversion/1
  Constant1/1 -> Bus Element Out7/1
  Constant/1 -> Bus Element Out5/1
  Gain/1 -> Signal Specification3/1
  Signal Specification3/1 -> Bus Element Out3/1, Bus Element Out4/1
  Clock/1 -> Gain/1
  Demux/3 -> Bus Element Out2/1
  Demux/2 -> Bus Element Out1/1
  Demux/1 -> Bus Element Out/1
  Bus Element In/1 -> Data Type Conversion1/1
  Constant2/1 -> Bus Element Out8/1
  Constant3/1 -> Bus Element Out9/1

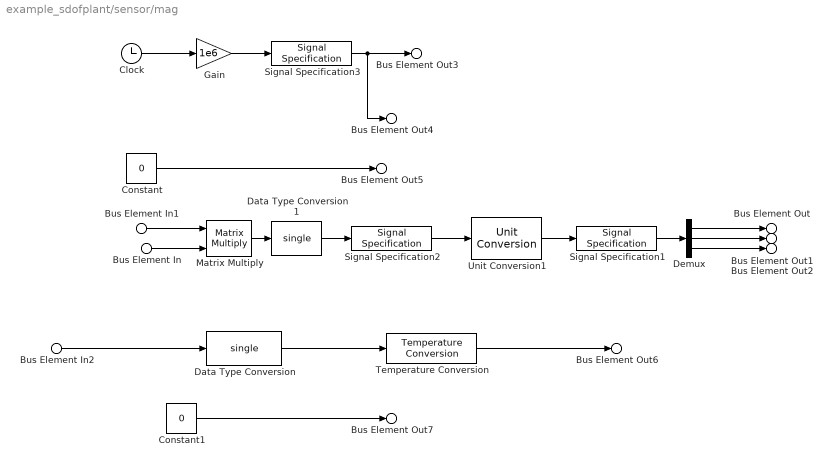
== system example_sdofplant/sensor/mag ==
  Bus Element In : Inport  PortName=state  Element=environ.magnetic.xyz
  Bus Element In2 : Inport  PortName=state  Element=environ.atmosphere.temperature
  Bus Element In1 : Inport  PortName=state  Element=aircraft.attitude.Rbe
  Clock : Clock
  Constant : Constant  Value=0  OutDataTypeStr=uint32
  Constant1 : Constant  Value=0  OutDataTypeStr=uint32
  Data Type Conversion : DataTypeConversion  OutDataTypeStr=single  SaturateOnIntegerOverflow=off  RndMeth=Floor
  Data Type Conversion1 : DataTypeConversion  OutDataTypeStr=single  SaturateOnIntegerOverflow=off  RndMeth=Floor
  Demux : Demux  Outputs=3
  Gain : Gain  Gain=1e6  OutDataTypeStr=uint64
  Matrix Multiply : Product  Multiplication=Matrix(*)
  Signal Specification1 : SignalSpecification  Unit=G
  Signal Specification2 : SignalSpecification  Unit=nT
  Signal Specification3 : SignalSpecification  Unit=µs
  Temperature Conversion : aerolibconvert2/Temperature Conversion  IU=K  OU=C
  Unit Conversion1 : UnitConversion
  Bus Element Out3 : Outport  PortName=mag  Element=timestamp
  Bus Element Out4 : Outport  PortName=mag  Element=timestamp_sample
  Bus Element Out5 : Outport  PortName=mag  Element=device_id
  Bus Element Out : Outport  PortName=mag  Element=x
  Bus Element Out1 : Outport  PortName=mag  Element=y
  Bus Element Out2 : Outport  PortName=mag  Element=z
  Bus Element Out6 : Outport  PortName=mag  Element=temperature
  Bus Element Out7 : Outport  PortName=mag  Element=error_count
  wires:
  Bus Element In/1 -> Matrix Multiply/2
  Bus Element In1/1 -> Matrix Multiply/1
  Matrix Multiply/1 -> Data Type Conversion1/1
  Demux/1 -> Bus Element Out/1
  Demux/2 -> Bus Element Out1/1
  Demux/3 -> Bus Element Out2/1
  Clock/1 -> Gain/1
  Signal Specification3/1 -> Bus Element Out4/1, Bus Element Out3/1
  Gain/1 -> Signal Specification3/1
  Constant/1 -> Bus Element Out5/1
  Constant1/1 -> Bus Element Out7/1
  Bus Element In2/1 -> Data Type Conversion/1
  Temperature Conversion/1 -> Bus Element Out6/1
  Data Type Conversion/1 -> Temperature Conversion/1
  Data Type Conversion1/1 -> Signal Specification2/1
  Signal Specification1/1 -> Demux/1
  Unit Conversion1/1 -> Signal Specification1/1
  Signal Specification2/1 -> Unit Conversion1/1

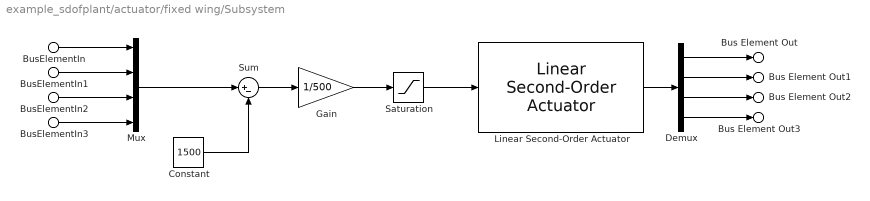
== system example_sdofplant/actuator/fixed wing/Subsystem ==
  BusElementIn : Inport  PortName=command  Element=pwm9
  BusElementIn1 : Inport  PortName=command  Element=pwm10
  BusElementIn2 : Inport  PortName=command  Element=pwm11
  BusElementIn3 : Inport  PortName=command  Element=pwm12
  Constant : Constant  Value=1500
  Demux : Demux
  Gain : Gain  Gain=1/500
  Linear Second-Order Actuator : aerolibactuator/Linear Second-Order Actuator  wn_fin=1  z_fin=0.3  fin_act_0=0  fin_act_vel=0
  Mux : Mux
  Saturation : Saturate  UpperLimit=1  LowerLimit=-1
  Sum : Sum  Inputs=|+-
  Bus Element Out : Outport  PortName=surface  Element=dla
  Bus Element Out1 : Outport  PortName=surface  Element=dra
  Bus Element Out2 : Outport  PortName=surface  Element=dlr
  Bus Element Out3 : Outport  PortName=surface  Element=drr
  wires:
  Mux/1 -> Sum/1
  Constant/1 -> Sum/2
  Gain/1 -> Saturation/1
  Sum/1 -> Gain/1
  Saturation/1 -> Linear Second-Order Actuator/1
  BusElementIn3/1 -> Mux/4
  BusElementIn1/1 -> Mux/2
  BusElementIn2/1 -> Mux/3
  BusElementIn/1 -> Mux/1
  Linear Second-Order Actuator/1 -> Demux/1
  Demux/1 -> Bus Element Out/1
  Demux/2 -> Bus Element Out1/1
  Demux/4 -> Bus Element Out3/1
  Demux/3 -> Bus Element Out2/1

== system example_sdofplant/actuator/fixed wing/Subsystem1 ==
  force : Inport
  moment : Inport  Port=2
  cog : Inport  Port=3
  pos : Inport  Port=4
  Out1 : Outport
  wires:
  force/1 -> Out1/1

== system example_sdofplant/actuator/fixed wing/basic ==
  Bus Element In1 : Inport  PortName=surface
  BusElementIn : Inport  Port=2  PortName=state  Element=aircraft.airdata.alpha
  Bus Element In2 : Inport  Port=2  PortName=state  Element=aircraft.airdata.bata
  2-D Lookup Table{,1..5} (6 alike) : Lookup_n-D  LookupTableObject=''  BreakpointsForDimension1=[1:2]  BreakpointsForDimension2=[1:2]  BreakpointsForDimension1FirstPoint=10  BreakpointsForDimension2FirstPoint=10  BreakpointsForDimension1Spacing=12  BreakpointsForDimension2Spacing=12  IndexSearchMethod=Evenly spaced points  Table=[4 5;16 19]  InterpMethod=Flat  DiagnosticForOutOfRangeInput=Error  InternalRulePriority=Speed  RndMeth=Simplest
      settings: InputPortMap=u0,u1
  Mux : Mux  Inputs=3
  Mux1 : Mux  Inputs=3
  Terminator : Terminator
  cxcycz : Outport
  clcmcn : Outport  Port=2
  wires:
  Bus Element In1/1 -> Terminator/1
  BusElementIn/1 -> 2-D Lookup Table5/1, 2-D Lookup Table4/1, 2-D Lookup Table3/1, 2-D Lookup Table2/1, 2-D Lookup Table1/1, 2-D Lookup Table/1
  Bus Element In2/1 -> 2-D Lookup Table/2, 2-D Lookup Table5/2, 2-D Lookup Table4/2, 2-D Lookup Table3/2, 2-D Lookup Table2/2, 2-D Lookup Table1/2
  2-D Lookup Table/1 -> Mux/1
  Mux/1 -> cxcycz/1
  2-D Lookup Table1/1 -> Mux/2
  2-D Lookup Table2/1 -> Mux/3
  2-D Lookup Table5/1 -> Mux1/3
  2-D Lookup Table4/1 -> Mux1/2
  2-D Lookup Table3/1 -> Mux1/1
  Mux1/1 -> clcmcn/1

== system example_sdofplant/actuator/fixed wing/landgear ==
  Bus Element In1 : Inport  PortName=surface
  BusElementIn : Inport  Port=2  PortName=state  Element=aircraft.airdata.alpha
  Bus Element In2 : Inport  Port=2  PortName=state  Element=aircraft.airdata.bata
  2-D Lookup Table{,1..5} (6 alike) : Lookup_n-D  LookupTableObject=''  BreakpointsForDimension1=[1:2]  BreakpointsForDimension2=[1:2]  BreakpointsForDimension1FirstPoint=10  BreakpointsForDimension2FirstPoint=10  BreakpointsForDimension1Spacing=12  BreakpointsForDimension2Spacing=12  IndexSearchMethod=Evenly spaced points  Table=[4 5;16 19]  InterpMethod=Flat  DiagnosticForOutOfRangeInput=Error  InternalRulePriority=Speed  RndMeth=Simplest
      settings: InputPortMap=u0,u1
  Mux : Mux  Inputs=3
  Mux1 : Mux  Inputs=3
  Terminator : Terminator
  cxcycz : Outport
  clcmcn : Outport  Port=2
  wires:
  Bus Element In1/1 -> Terminator/1
  BusElementIn/1 -> 2-D Lookup Table5/1, 2-D Lookup Table4/1, 2-D Lookup Table3/1, 2-D Lookup Table2/1, 2-D Lookup Table1/1, 2-D Lookup Table/1
  Bus Element In2/1 -> 2-D Lookup Table/2, 2-D Lookup Table5/2, 2-D Lookup Table4/2, 2-D Lookup Table3/2, 2-D Lookup Table2/2, 2-D Lookup Table1/2
  2-D Lookup Table/1 -> Mux/1
  Mux/1 -> cxcycz/1
  2-D Lookup Table1/1 -> Mux/2
  2-D Lookup Table2/1 -> Mux/3
  2-D Lookup Table5/1 -> Mux1/3
  2-D Lookup Table4/1 -> Mux1/2
  2-D Lookup Table3/1 -> Mux1/1
  Mux1/1 -> clcmcn/1

== system example_sdofplant/actuator/fixed wing/left aileron ==
  Bus Element In1 : Inport  PortName=surface  Element=signal1
  state : Inport  Port=2
  Out1 : Outport
  Out2 : Outport  Port=2

== system example_sdofplant/actuator/fixed wing/left rudder ==
  Bus Element In1 : Inport  PortName=surface  Element=signal1
  state : Inport  Port=2
  Out1 : Outport
  Out2 : Outport  Port=2

== system example_sdofplant/actuator/fixed wing/right aileron ==
  Bus Element In1 : Inport  PortName=surface  Element=signal1
  state : Inport  Port=2
  Out1 : Outport
  Out2 : Outport  Port=2

== system example_sdofplant/actuator/fixed wing/right rudder ==
  Bus Element In1 : Inport  PortName=surface  Element=signal1
  state : Inport  Port=2
  Out1 : Outport
  Out2 : Outport  Port=2

== system example_sdofplant/sensor/gps/posix time ==
  Clock : Clock
  Constant : Constant  Value=convertTo(datetime('now','TimeZone','UTC'),'posixtime')
  Gain : Gain  Gain=1e6  OutDataTypeStr=uint64
  Sum : Sum  Inputs=|++
  utc : Outport  Unit=µs
  wires:
  Clock/1 -> Sum/1
  Sum/1 -> Gain/1
  Constant/1 -> Sum/2
  Gain/1 -> utc/1
